simulink model "double_integrator_sim"  (R2023a)
settings: Solver=VariableStepAuto  StartTime=0.0  StopTime=200  FixedStep=0.0001  RelTol=1e-9
values from neighbouring files (symbols this model uses):
  framePeriod_s = 1/frameRate_hz    (= 0.02)    [autocode_setup.m]    (also in setup.m)
undefined symbols (not defined in the file or in its folder): Aircraft, magnitude
libraries: slpidlib x15, simulink x12, dspmathops x2, shared6dof x1, sharedtransform x1
(part 2 of 3)

== system double_integrator_sim/WAYPOINT CONTROLLER1/WP_NAV/Subsystem ==
  Sys_input : Inport
  tar_pos : Inport  Port=2
  max_v_z_mps : Inport  Port=3
  Bus Selector : BusSelector  OutputSignals=StateEstData.aux_ins.ned_pos_m
  Cast To Single : DataTypeConversion  OutDataTypeStr=single  SaturateOnIntegerOverflow=off  RndMeth=Floor
  Selector : Selector  InputPortWidth=3  IndexOptions=Index vector (dialog)  Indices=3  OutputSizes=1
  Selector1 : Selector  InputPortWidth=3  IndexOptions=Index vector (dialog)  Indices=3  OutputSizes=1
  Vertical position controller1 : Subsystem
  ve_z_cmd_mps : Outport
  wires:
  Vertical position controller1/1(ve_z_cmd_mps) -> ve_z_cmd_mps/1  "ve_z_cmd_mps"
  tar_pos/1 -> Selector/1
  Sys_input/1 -> Bus Selector/1
  Bus Selector/1 -> Selector1/1  "<ned_pos_m>"
  Selector1/1 -> Cast To Single/1
  max_v_z_mps/1 -> Vertical position controller1/3(max_v_z_mps)
  Selector/1 -> Vertical position controller1/2(tar_z)
  Cast To Single/1 -> Vertical position controller1/1(cur_alt)

== system double_integrator_sim/WAYPOINT CONTROLLER1/WP_NAV/Vertical position controller ==
  Sys_input : Inport
  max_v_z_mps : Inport  Port=2
  cur_target_pos_m : Inport  Port=3
  Bus Selector6 : BusSelector  OutputSignals=Navigation Filter Data.bfs_ekf.ned_pos_m
  Selector1 : Selector  InputPortWidth=3  IndexOptions=Index vector (dialog)  Indices=3  OutputSizes=1
  select_cur_z : Selector  InputPortWidth=3  IndexOptions=Index vector (dialog)  Indices=3  OutputSizes=1
  vertical_position_controller : Subsystem
  ve_z_cmd_mps : Outport
  wires:
  Sys_input/1 -> Bus Selector6/1
  Bus Selector6/1 -> select_cur_z/1  "<ned_pos_m>"
  vertical_position_controller/1(ve_z_cmd) -> ve_z_cmd_mps/1
  Selector1/1 -> vertical_position_controller/1(target_z_m)  "target_z"
  select_cur_z/1 -> vertical_position_controller/2(cur_z_m)
  cur_target_pos_m/1 -> Selector1/1
  max_v_z_mps/1 -> vertical_position_controller/3(max_v_z_mps)

== system double_integrator_sim/WAYPOINT CONTROLLER1/WP_NAV/heading_controller ==
  Sys_input : Inport
  cur_target_heading_rad : Inport  Port=2
  Bus Selector4 : BusSelector  OutputSignals=Navigation Filter Data.bfs_ekf.heading_rad
  heading_controller : Subsystem
  yaw_rate_cmd_radps : Outport
  wires:
  Sys_input/1 -> Bus Selector4/1
  cur_target_heading_rad/1 -> heading_controller/1(heading_cmd_rad)
  Bus Selector4/1 -> heading_controller/2(<heading_rad>)  "<heading_rad>"
  heading_controller/1(yaw_rate_cmd) -> yaw_rate_cmd_radps/1

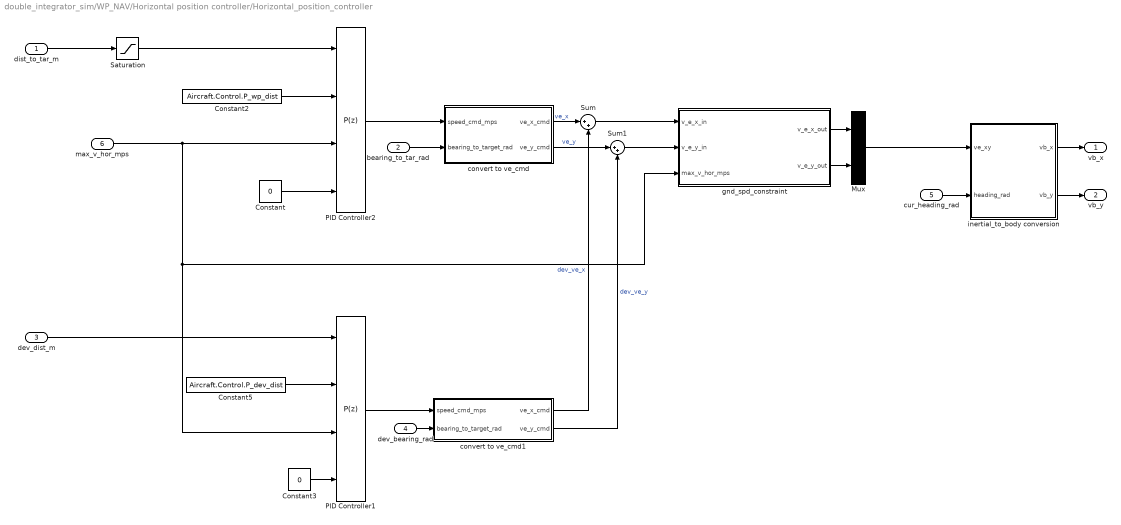
== system double_integrator_sim/WP_NAV/Horizontal position controller/Horizontal_position_controller ==
  dist_to_tar_m : Inport
  bearing_to_tar_rad : Inport  Port=2
  dev_dist_m : Inport  Port=3
  dev_bearing_rad : Inport  Port=4
  cur_heading_rad : Inport  Port=5
  max_v_hor_mps : Inport  Port=6
  Constant : Constant  Value=0  OutDataTypeStr=single
  Constant2 : Constant  Value=Aircraft.Control.P_wp_dist  OutDataTypeStr=single
  Constant3 : Constant  Value=0  OutDataTypeStr=single
  Constant5 : Constant  Value=Aircraft.Control.P_dev_dist  OutDataTypeStr=single
  Mux : Mux  Inputs=2
  PID Controller1 : slpidlib/PID Controller  Controller=P  Form=Parallel  TimeDomain=Discrete-time  UseExternalTs=off  SampleTime=framePeriod_s  IntegratorMethod=Forward Euler  FilterMethod=Forward Euler  ControllerParametersSource=external  P=0.335  I=0.005  UseKiTs=off  D=0  N=100  UseFilter=off  TunerSelectOption=Transfer Function Based (PID Tuner App)  InitialConditionSource=internal  InitialConditionForIntegrator=0  InitialConditionForFilter=0  DifferentiatorICPrevScaledInput=0  ExternalReset=none  TrackingMode=off  Kt=1  LimitOutput=on  SatLimitsSource=external  UpperSaturationLimit=inf  LowerSaturationLimit=-inf  LinearizeAsGain=off  AntiWindupMode=clamping  Kb=1  LimitIntegrator=off  UpperIntegratorSaturationLimit=inf  LowerIntegratorSaturationLimit=-inf  POutMin=[]  POutMax=[]  IOutMin=[]  IOutMax=[]  DOutMin=[]  DOutMax=[]  NOutMin=[]  NOutMax=[]  SumOutMin=[]  SumOutMax=[]  SaturationOutMin=[]  SaturationOutMax=[]  PParamMin=[]  PParamMax=[]  IParamMin=[]  IParamMax=[]  DParamMin=[]  DParamMax=[]  NParamMin=[]  NParamMax=[]  KbParamMin=[]  KbParamMax=[]  KtParamMin=[]  KtParamMax=[]  KbOutMin=[]  KbOutMax=[]  KtOutMin=[]  KtOutMax=[]  IntegratorOutMin=[]  IntegratorOutMax=[]  FilterOutMin=[]  FilterOutMax=[]  SumI1OutMin=[]  SumI1OutMax=[]  SumI2OutMin=[]  SumI2OutMax=[]  SumI3OutMin=[]  SumI3OutMax=[]  SumI4OutMin=[]  SumI4OutMax=[]  SumDOutMin=[]  SumDOutMax=[]  DifferentiatorOutMin=[]  DifferentiatorOutMax=[]  FilterDiffOutCoefMin=[]  FilterDiffOutCoefMax=[]  ReciprocalOutMin=[]  ReciprocalOutMax=[]  SumDenOutMin=[]  SumDenOutMax=[]  SumNumOutMin=[]  SumNumOutMax=[]  DivideOutMin=[]  DivideOutMax=[]  UdiffTsProdOutMin=[]  UdiffTsProdOutMax=[]  NTsProdOutMin=[]  NTsProdOutMax=[]  UintegralTsProdOutMin=[]  UintegralTsProdOutMax=[]  UngainTsProdOutMin=[]  UngainTsProdOutMax=[]  ClampingZeroOutDataTypeStr=Inherit: Inherit via back propagation  ClampingZeroOutMin=[]  ClampingZeroOutMax=[]  FilterDenConstantOutDataTypeStr=Inherit: Inherit via back propagation  FilterDenConstantOutMin=[]  FilterDenConstantOutMax=[]  PCopyOutDataTypeStr=Inherit: Inherit via back propagation  PCopyOutMin=[]  PCopyOutMax=[]  NCopyOutDataTypeStr=Inherit: Inherit via back propagation  NCopyOutMin=[]  NCopyOutMax=[]  IntegratorContinuousStateAttributes=''  IntegratorStateMustResolveToSignalObject=off  IntegratorRTWStateStorageClass=Auto  FilterContinuousStateAttributes=''  FilterStateMustResolveToSignalObject=off  FilterRTWStateStorageClass=Auto  ParallelPVariant=ExternalParameters  IdealPVariant=Disabled  IVariant=Disabled  DVariant=Disabled  IntegratorVariant=Disabled  SatVariant=External  AWVariant=Disabled  PCopyVariant=Disabled  TRVariant=Disabled  FdbkBlocksVariant=Forward  IdealPFdbkVariant=Disabled  SatFdbkVariant=Disabled  DerivativeFilterVariant=Disabled  NVariant=Disabled  NCopyVariant=Disabled_SignalSpec  FilterICVariant=Disabled  IntegratorICVariant=Disabled  ExternalResetVariant=Disabled  TRSumVariant=Passthrough  SumFdbkVariant=Disabled  SumVariant=Passthrough_P  TsampFilterVariant=InternalTs  TsampNgainVariant=Passthrough  TsampIntegralVariant=Disabled_SignalSpec  ExternalSaturationOutDataTypeStr=Inherit: Same as second input
  PID Controller2 : slpidlib/PID Controller  Controller=P  Form=Parallel  TimeDomain=Discrete-time  UseExternalTs=off  SampleTime=framePeriod_s  IntegratorMethod=Forward Euler  FilterMethod=Forward Euler  ControllerParametersSource=external  P=0.335  I=0.005  UseKiTs=off  D=0  N=100  UseFilter=off  TunerSelectOption=Transfer Function Based (PID Tuner App)  InitialConditionSource=internal  InitialConditionForIntegrator=0  InitialConditionForFilter=0  DifferentiatorICPrevScaledInput=0  ExternalReset=none  TrackingMode=off  Kt=1  LimitOutput=on  SatLimitsSource=external  UpperSaturationLimit=inf  LowerSaturationLimit=-inf  LinearizeAsGain=off  AntiWindupMode=clamping  Kb=1  LimitIntegrator=off  UpperIntegratorSaturationLimit=inf  LowerIntegratorSaturationLimit=-inf  POutMin=[]  POutMax=[]  IOutMin=[]  IOutMax=[]  DOutMin=[]  DOutMax=[]  NOutMin=[]  NOutMax=[]  SumOutMin=[]  SumOutMax=[]  SaturationOutMin=[]  SaturationOutMax=[]  PParamMin=[]  PParamMax=[]  IParamMin=[]  IParamMax=[]  DParamMin=[]  DParamMax=[]  NParamMin=[]  NParamMax=[]  KbParamMin=[]  KbParamMax=[]  KtParamMin=[]  KtParamMax=[]  KbOutMin=[]  KbOutMax=[]  KtOutMin=[]  KtOutMax=[]  IntegratorOutMin=[]  IntegratorOutMax=[]  FilterOutMin=[]  FilterOutMax=[]  SumI1OutMin=[]  SumI1OutMax=[]  SumI2OutMin=[]  SumI2OutMax=[]  SumI3OutMin=[]  SumI3OutMax=[]  SumI4OutMin=[]  SumI4OutMax=[]  SumDOutMin=[]  SumDOutMax=[]  DifferentiatorOutMin=[]  DifferentiatorOutMax=[]  FilterDiffOutCoefMin=[]  FilterDiffOutCoefMax=[]  ReciprocalOutMin=[]  ReciprocalOutMax=[]  SumDenOutMin=[]  SumDenOutMax=[]  SumNumOutMin=[]  SumNumOutMax=[]  DivideOutMin=[]  DivideOutMax=[]  UdiffTsProdOutMin=[]  UdiffTsProdOutMax=[]  NTsProdOutMin=[]  NTsProdOutMax=[]  UintegralTsProdOutMin=[]  UintegralTsProdOutMax=[]  UngainTsProdOutMin=[]  UngainTsProdOutMax=[]  ClampingZeroOutDataTypeStr=Inherit: Inherit via back propagation  ClampingZeroOutMin=[]  ClampingZeroOutMax=[]  FilterDenConstantOutDataTypeStr=Inherit: Inherit via back propagation  FilterDenConstantOutMin=[]  FilterDenConstantOutMax=[]  PCopyOutDataTypeStr=Inherit: Inherit via back propagation  PCopyOutMin=[]  PCopyOutMax=[]  NCopyOutDataTypeStr=Inherit: Inherit via back propagation  NCopyOutMin=[]  NCopyOutMax=[]  IntegratorContinuousStateAttributes=''  IntegratorStateMustResolveToSignalObject=off  IntegratorRTWStateStorageClass=Auto  FilterContinuousStateAttributes=''  FilterStateMustResolveToSignalObject=off  FilterRTWStateStorageClass=Auto  ParallelPVariant=ExternalParameters  IdealPVariant=Disabled  IVariant=Disabled  DVariant=Disabled  IntegratorVariant=Disabled  SatVariant=External  AWVariant=Disabled  PCopyVariant=Disabled  TRVariant=Disabled  FdbkBlocksVariant=Forward  IdealPFdbkVariant=Disabled  SatFdbkVariant=Disabled  DerivativeFilterVariant=Disabled  NVariant=Disabled  NCopyVariant=Disabled_SignalSpec  FilterICVariant=Disabled  IntegratorICVariant=Disabled  ExternalResetVariant=Disabled  TRSumVariant=Passthrough  SumFdbkVariant=Disabled  SumVariant=Passthrough_P  TsampFilterVariant=InternalTs  TsampNgainVariant=Passthrough  TsampIntegralVariant=Disabled_SignalSpec  ExternalSaturationOutDataTypeStr=Inherit: Same as second input
  Saturation : Saturate  UpperLimit=1  LowerLimit=0
  Sum : Sum  Inputs=|++
  Sum1 : Sum  Inputs=|++
  convert to ve_cmd : Subsystem
  convert to ve_cmd1 : Subsystem
  "gnd_spd_constraint " : Subsystem
  inertial_to_body conversion : Subsystem
  vb_x : Outport
  vb_y : Outport  Port=2
  wires:
  Constant2/1 -> PID Controller2/2
  bearing_to_tar_rad/1 -> convert to ve_cmd/2(bearing_to_target_rad)
  Mux/1 -> inertial_to_body conversion/1(ve_xy)
  Constant/1 -> PID Controller2/4
  Saturation/1 -> PID Controller2/1
  dist_to_tar_m/1 -> Saturation/1
  cur_heading_rad/1 -> inertial_to_body conversion/2(heading_rad)
  PID Controller2/1 -> convert to ve_cmd/1(speed_cmd_mps)
  inertial_to_body conversion/1(vb_x) -> vb_x/1
  inertial_to_body conversion/2(vb_y) -> vb_y/1
  PID Controller1/1 -> convert to ve_cmd1/1(speed_cmd_mps)
  dev_bearing_rad/1 -> convert to ve_cmd1/2(bearing_to_target_rad)
  dev_dist_m/1 -> PID Controller1/1
  Constant3/1 -> PID Controller1/4
  max_v_hor_mps/1 -> PID Controller1/3, "gnd_spd_constraint "/3(max_v_hor_mps), PID Controller2/3
  convert to ve_cmd/1(ve_x_cmd) -> Sum/1  "ve_x"
  convert to ve_cmd/2(ve_y_cmd) -> Sum1/1  "ve_y"
  convert to ve_cmd1/1(ve_x_cmd) -> Sum/2  "dev_ve_x"
  convert to ve_cmd1/2(ve_y_cmd) -> Sum1/2  "dev_ve_y"
  Sum1/1 -> "gnd_spd_constraint "/2(v_e_y_in)
  Sum/1 -> "gnd_spd_constraint "/1(v_e_x_in)
  "gnd_spd_constraint "/1(v_e_x_out) -> Mux/1
  "gnd_spd_constraint "/2(v_e_y_out) -> Mux/2
  Constant5/1 -> PID Controller1/2

== system double_integrator_sim/WP_NAV/Horizontal position controller/horizontal_error_calculation  ==
  target_pos_m : Inport
  cur_pos_m : Inport  Port=2
  Atan2 : Trigonometry  Operator=atan2
  Cast To Single : DataTypeConversion  OutDataTypeStr=single  SaturateOnIntegerOverflow=off  RndMeth=Floor
  Cast To Single1 : DataTypeConversion  OutDataTypeStr=single  SaturateOnIntegerOverflow=off  RndMeth=Floor
  Demux2 : Demux  Outputs=2
  MatrixMultiply : Product  Multiplication=Matrix(*)
  Selector : Selector  InputPortWidth=3  IndexOptions=Index vector (dialog)  Indices=[1 2]  OutputSizes=1
  Sqrt : Sqrt
  Subtract : Sum  Inputs=+-
  Transpose : Math  Operator=transpose
  dist_to_target_m : Outport
  bearing_to_tar_rad : Outport  Port=2
  wires:
  target_pos_m/1 -> Subtract/1
  cur_pos_m/1 -> Subtract/2
  Selector/1 -> Demux2/1, MatrixMultiply/2, Transpose/1
  Atan2/1 -> Cast To Single1/1
  Subtract/1 -> Selector/1
  Demux2/2 -> Atan2/1
  Transpose/1 -> MatrixMultiply/1
  MatrixMultiply/1 -> Sqrt/1
  Demux2/1 -> Atan2/2
  Sqrt/1 -> Cast To Single/1
  Cast To Single/1 -> dist_to_target_m/1
  Cast To Single1/1 -> bearing_to_tar_rad/1

== system double_integrator_sim/WP_NAV/Subsystem/Vertical position controller1 ==
  cur_alt : Inport
  tar_z : Inport  Port=2
  max_v_z_mps : Inport  Port=3
  Altitude PID : slpidlib/PID Controller  Controller=P  Form=Ideal  TimeDomain=Discrete-time  UseExternalTs=off  SampleTime=framePeriod_s  IntegratorMethod=Forward Euler  FilterMethod=Forward Euler  ControllerParametersSource=external  P=0  I=0  UseKiTs=off  D=0  N=100  UseFilter=off  TunerSelectOption=Frequency Response Based  ZeroCross=off  InitialConditionSource=internal  InitialConditionForIntegrator=0  InitialConditionForFilter=0  DifferentiatorICPrevScaledInput=0  ExternalReset=either  TrackingMode=off  Kt=1  LimitOutput=on  SatLimitsSource=external  UpperSaturationLimit=Aircraft.Control.v_z_max  LowerSaturationLimit=-Aircraft.Control.v_z_max  LinearizeAsGain=on  AntiWindupMode=clamping  Kb=1  LimitIntegrator=off  UpperIntegratorSaturationLimit=inf  LowerIntegratorSaturationLimit=-inf  POutMin=[]  POutMax=[]  IOutMin=[]  IOutMax=[]  DOutMin=[]  DOutMax=[]  NOutMin=[]  NOutMax=[]  SumOutMin=[]  SumOutMax=[]  SaturationOutMin=[]  SaturationOutMax=[]  PParamMin=[]  PParamMax=[]  IParamMin=[]  IParamMax=[]  DParamMin=[]  DParamMax=[]  NParamMin=[]  NParamMax=[]  KbParamMin=[]  KbParamMax=[]  KtParamMin=[]  KtParamMax=[]  KbOutMin=[]  KbOutMax=[]  KtOutMin=[]  KtOutMax=[]  IntegratorOutMin=[]  IntegratorOutMax=[]  FilterOutMin=[]  FilterOutMax=[]  SumI1OutMin=[]  SumI1OutMax=[]  SumI2OutMin=[]  SumI2OutMax=[]  SumI3OutMin=[]  SumI3OutMax=[]  SumI4OutMin=[]  SumI4OutMax=[]  SumDOutMin=[]  SumDOutMax=[]  DifferentiatorOutMin=[]  DifferentiatorOutMax=[]  FilterDiffOutCoefMin=[]  FilterDiffOutCoefMax=[]  ReciprocalOutMin=[]  ReciprocalOutMax=[]  SumDenOutMin=[]  SumDenOutMax=[]  SumNumOutMin=[]  SumNumOutMax=[]  DivideOutMin=[]  DivideOutMax=[]  UdiffTsProdOutMin=[]  UdiffTsProdOutMax=[]  NTsProdOutMin=[]  NTsProdOutMax=[]  UintegralTsProdOutMin=[]  UintegralTsProdOutMax=[]  UngainTsProdOutMin=[]  UngainTsProdOutMax=[]  ClampingZeroOutDataTypeStr=Inherit: Inherit via back propagation  ClampingZeroOutMin=[]  ClampingZeroOutMax=[]  FilterDenConstantOutDataTypeStr=Inherit: Inherit via back propagation  FilterDenConstantOutMin=[]  FilterDenConstantOutMax=[]  PCopyOutDataTypeStr=Inherit: Inherit via back propagation  PCopyOutMin=[]  PCopyOutMax=[]  NCopyOutDataTypeStr=Inherit: Inherit via back propagation  NCopyOutMin=[]  NCopyOutMax=[]  IntegratorContinuousStateAttributes=''  IntegratorStateMustResolveToSignalObject=off  IntegratorRTWStateStorageClass=Auto  FilterContinuousStateAttributes=''  FilterStateMustResolveToSignalObject=off  FilterRTWStateStorageClass=Auto  ParallelPVariant=ExternalParameters  IdealPVariant=Disabled  IVariant=Disabled  DVariant=Disabled  IntegratorVariant=Disabled  SatVariant=External  AWVariant=Disabled  PCopyVariant=Disabled  TRVariant=Disabled  FdbkBlocksVariant=Forward  IdealPFdbkVariant=Disabled  SatFdbkVariant=Disabled  DerivativeFilterVariant=Disabled  NVariant=Disabled  NCopyVariant=Disabled_SignalSpec  FilterICVariant=Disabled  IntegratorICVariant=Disabled  ExternalResetVariant=Disabled  TRSumVariant=Passthrough  SumFdbkVariant=Disabled  SumVariant=Passthrough_P  TsampFilterVariant=InternalTs  TsampNgainVariant=Passthrough  TsampIntegralVariant=Disabled_SignalSpec  ExternalSaturationOutDataTypeStr=Inherit: Same as second input
  Constant3 : Constant  Value=0.1  OutDataTypeStr=single
  Gain : Gain  Gain=-1
  Scope : Scope  NumInputPorts=3
  Sum3 : Sum  Inputs=|+-
  ve_z_cmd_mps : Outport
  wires:
  Altitude PID/1 -> Scope/3, ve_z_cmd_mps/1
  tar_z/1 -> Scope/1, Sum3/1  "target_z"
  cur_alt/1 -> Scope/2, Sum3/2
  Sum3/1 -> Altitude PID/1
  Constant3/1 -> Altitude PID/2
  max_v_z_mps/1 -> Gain/1, Altitude PID/3
  Gain/1 -> Altitude PID/4

== system double_integrator_sim/WP_NAV/Vertical position controller/vertical_position_controller ==
  target_z_m : Inport
  cur_z_m : Inport  Port=2
  max_v_z_mps : Inport  Port=3
  Altitude PID : slpidlib/PID Controller  Controller=PI  Form=Ideal  TimeDomain=Discrete-time  UseExternalTs=off  SampleTime=framePeriod_s  IntegratorMethod=Forward Euler  FilterMethod=Forward Euler  ControllerParametersSource=external  P=0  I=0  UseKiTs=off  D=0  N=100  UseFilter=off  TunerSelectOption=Frequency Response Based  ZeroCross=off  InitialConditionSource=internal  InitialConditionForIntegrator=0  InitialConditionForFilter=0  DifferentiatorICPrevScaledInput=0  ExternalReset=none  TrackingMode=off  Kt=1  LimitOutput=on  SatLimitsSource=external  UpperSaturationLimit=Aircraft.Control.v_z_up_max  LowerSaturationLimit=-Aircraft.Control.v_z_down_max  LinearizeAsGain=on  AntiWindupMode=clamping  Kb=1  POutMin=[]  POutMax=[]  IOutMin=[]  IOutMax=[]  DOutMin=[]  DOutMax=[]  NOutMin=[]  NOutMax=[]  SumOutMin=[]  SumOutMax=[]  SaturationOutMin=[]  SaturationOutMax=[]  PParamMin=[]  PParamMax=[]  IParamMin=[]  IParamMax=[]  DParamMin=[]  DParamMax=[]  NParamMin=[]  NParamMax=[]  KbParamMin=[]  KbParamMax=[]  KtParamMin=[]  KtParamMax=[]  KbOutMin=[]  KbOutMax=[]  KtOutMin=[]  KtOutMax=[]  IntegratorOutMin=[]  IntegratorOutMax=[]  FilterOutMin=[]  FilterOutMax=[]  SumI1OutMin=[]  SumI1OutMax=[]  SumI2OutMin=[]  SumI2OutMax=[]  SumI3OutMin=[]  SumI3OutMax=[]  SumI4OutMin=[]  SumI4OutMax=[]  SumDOutMin=[]  SumDOutMax=[]  DifferentiatorOutMin=[]  DifferentiatorOutMax=[]  FilterDiffOutCoefMin=[]  FilterDiffOutCoefMax=[]  ReciprocalOutMin=[]  ReciprocalOutMax=[]  SumDenOutMin=[]  SumDenOutMax=[]  SumNumOutMin=[]  SumNumOutMax=[]  DivideOutMin=[]  DivideOutMax=[]  UdiffTsProdOutMin=[]  UdiffTsProdOutMax=[]  NTsProdOutMin=[]  NTsProdOutMax=[]  UintegralTsProdOutMin=[]  UintegralTsProdOutMax=[]  UngainTsProdOutMin=[]  UngainTsProdOutMax=[]  IntegratorContinuousStateAttributes=''  IntegratorStateMustResolveToSignalObject=off  IntegratorRTWStateStorageClass=Auto  FilterContinuousStateAttributes=''  FilterStateMustResolveToSignalObject=off  FilterRTWStateStorageClass=Auto  ParallelPVariant=Passthrough  IdealPVariant=ExternalParameters  IVariant=ExternalParameters  DVariant=Disabled  IntegratorVariant=Discrete  SatVariant=External  AWVariant=DiscClampingIdeal  PCopyVariant=ExternalParamsIdeal  TRVariant=Disabled  FdbkBlocksVariant=Forward  IdealPFdbkVariant=Disabled  SatFdbkVariant=Disabled  DerivativeFilterVariant=Disabled  NVariant=Disabled  NCopyVariant=Disabled_SignalSpec  FilterICVariant=Disabled  IntegratorICVariant=InternalICs  ExternalResetVariant=Disabled  TRSumVariant=Passthrough  SumFdbkVariant=Disabled  SumVariant=Sum_PI  TsampFilterVariant=InternalTs  TsampNgainVariant=Passthrough  TsampIntegralVariant=Passthrough  ExternalSaturationOutDataTypeStr=Inherit: Same as second input  aMode=0
  Constant : Constant  Value=Aircraft.Control.v_z_up_max  OutDataTypeStr=single
  Constant1 : Constant  Value=Aircraft.Control.v_z_down_max  OutDataTypeStr=single
  Gain : Gain  Gain=-1
  Min : MinMax  Inputs=2
  P_alt : Constant  Value=Aircraft.Control.P_alt  OutDataTypeStr=single
  P_alt1 : Constant  Value=Aircraft.Control.I_alt  OutDataTypeStr=single
  Sum3 : Sum  Inputs=|+-
  ve_z_cmd : Outport
  wires:
  P_alt/1 -> Altitude PID/2
  Sum3/1 -> Altitude PID/1
  max_v_z_mps/1 -> Min/1
  Constant/1 -> Min/2
  Constant1/1 -> Altitude PID/4
  Min/1 -> Gain/1
  Gain/1 -> Altitude PID/5
  P_alt1/1 -> Altitude PID/3
  Altitude PID/1 -> ve_z_cmd/1
  target_z_m/1 -> Sum3/1
  cur_z_m/1 -> Sum3/2

== system double_integrator_sim/WP_NAV/heading_controller/heading_controller ==
  heading_cmd_rad : Inport
  <heading_rad> : Inport  Port=2
  D_heading : Constant  Value=Aircraft.Control.D_heading  OutDataTypeStr=single
  Discrete Derivative : simulink/Discrete/Discrete Derivative  gainval=1.0  ICPrevScaledInput=0.0  OutMin=[]  OutMax=[]  OutDataType=fixdt(1, 16)  OutScaling=2^-10  DoSatur=off
  I_heading : Constant  Value=Aircraft.Control.I_heading  OutDataTypeStr=single
  PID Controller2 : slpidlib/PID Controller  Controller=PI  Form=Ideal  TimeDomain=Discrete-time  UseExternalTs=off  SampleTime=framePeriod_s  IntegratorMethod=Forward Euler  FilterMethod=Forward Euler  ControllerParametersSource=external  P=1.85  I=0.01  UseKiTs=off  D=0  N=100  UseFilter=off  TunerSelectOption=Transfer Function Based (PID Tuner App)  InitialConditionSource=internal  InitialConditionForIntegrator=0  InitialConditionForFilter=0  DifferentiatorICPrevScaledInput=0  ExternalReset=none  TrackingMode=off  Kt=1  LimitOutput=on  SatLimitsSource=internal  UpperSaturationLimit=inf  LowerSaturationLimit=-inf  LinearizeAsGain=on  AntiWindupMode=clamping  Kb=2  POutMin=[]  POutMax=[]  IOutMin=[]  IOutMax=[]  DOutMin=[]  DOutMax=[]  NOutMin=[]  NOutMax=[]  SumOutMin=[]  SumOutMax=[]  SaturationOutMin=[]  SaturationOutMax=[]  PParamMin=[]  PParamMax=[]  IParamMin=[]  IParamMax=[]  DParamMin=[]  DParamMax=[]  NParamMin=[]  NParamMax=[]  KbParamMin=[]  KbParamMax=[]  KtParamMin=[]  KtParamMax=[]  KbOutMin=[]  KbOutMax=[]  KtOutMin=[]  KtOutMax=[]  IntegratorOutMin=[]  IntegratorOutMax=[]  FilterOutMin=[]  FilterOutMax=[]  SumI1OutMin=[]  SumI1OutMax=[]  SumI2OutMin=[]  SumI2OutMax=[]  SumI3OutMin=[]  SumI3OutMax=[]  SumI4OutMin=[]  SumI4OutMax=[]  SumDOutMin=[]  SumDOutMax=[]  DifferentiatorOutMin=[]  DifferentiatorOutMax=[]  FilterDiffOutCoefMin=[]  FilterDiffOutCoefMax=[]  ReciprocalOutMin=[]  ReciprocalOutMax=[]  SumDenOutMin=[]  SumDenOutMax=[]  SumNumOutMin=[]  SumNumOutMax=[]  DivideOutMin=[]  DivideOutMax=[]  UdiffTsProdOutMin=[]  UdiffTsProdOutMax=[]  NTsProdOutMin=[]  NTsProdOutMax=[]  UintegralTsProdOutMin=[]  UintegralTsProdOutMax=[]  UngainTsProdOutMin=[]  UngainTsProdOutMax=[]  IntegratorContinuousStateAttributes=''  IntegratorStateMustResolveToSignalObject=off  IntegratorRTWStateStorageClass=Auto  FilterContinuousStateAttributes=''  FilterStateMustResolveToSignalObject=off  FilterRTWStateStorageClass=Auto  ParallelPVariant=Passthrough  IdealPVariant=ExternalParameters  IVariant=ExternalParameters  DVariant=Disabled  IntegratorVariant=Discrete  SatVariant=Enabled  AWVariant=DiscClampingIdeal  PCopyVariant=ExternalParamsIdeal  TRVariant=Disabled  FdbkBlocksVariant=Forward  IdealPFdbkVariant=Disabled  SatFdbkVariant=Disabled  DerivativeFilterVariant=Disabled  NVariant=Disabled  NCopyVariant=Disabled_SignalSpec  FilterICVariant=Disabled  IntegratorICVariant=InternalICs  ExternalResetVariant=Disabled  TRSumVariant=Passthrough  SumFdbkVariant=Disabled  SumVariant=Sum_PI  TsampFilterVariant=InternalTs  TsampNgainVariant=Passthrough  TsampIntegralVariant=Passthrough  ExternalSaturationOutDataTypeStr=Inherit: Same as second input  aMode=0
  P_heading : Constant  Value=Aircraft.Control.P_heading  OutDataTypeStr=single
  Product : Product
  Saturation : Saturate  UpperLimit=Aircraft.Control.yaw_rate_max  LowerLimit=-Aircraft.Control.yaw_rate_max
  Sum : Sum  Inputs=|+-
  heading_error : Subsystem
  yaw_rate_cmd : Outport
  wires:
  P_heading/1 -> PID Controller2/2
  heading_cmd_rad/1 -> heading_error/1(heading_cmd_rad)
  I_heading/1 -> PID Controller2/3
  <heading_rad>/1 -> Discrete Derivative/1, heading_error/2(heading_rad)
  Saturation/1 -> yaw_rate_cmd/1
  heading_error/1(heading_error_rad) -> PID Controller2/1
  Discrete Derivative/1 -> Product/1
  D_heading/1 -> Product/2
  PID Controller2/1 -> Sum/1
  Sum/1 -> Saturation/1
  Product/1 -> Sum/2

== system double_integrator_sim/POS_HOLD CONTROLLER/Horizontal speed controller/Subsystem/roll_D_DLPF ==
  raw_val : Inport
  freq_cut : Inport  Port=2
  Cast To Single : DataTypeConversion  OutDataTypeStr=single  SaturateOnIntegerOverflow=off  RndMeth=Floor
  Constant : Constant  Value=50  OutDataTypeStr=single
  MATLAB Function : MATLAB Function  TreatAsAtomicUnit=on
  Unit Delay : UnitDelay  SampleTime=-1  HasFrameUpgradeWarning=on
  filtered_val : Outport
  wires:
  freq_cut/1 -> MATLAB Function/3(freq_cut)
  MATLAB Function/1(filtered_val) -> Unit Delay/1, filtered_val/1
  Unit Delay/1 -> Cast To Single/1
  raw_val/1 -> MATLAB Function/2(raw_val)
  Constant/1 -> MATLAB Function/4(samp_freq)
  Cast To Single/1 -> MATLAB Function/1(prev_val)

== system double_integrator_sim/POS_HOLD CONTROLLER/Horizontal speed controller/Subsystem/roll_D_DLPF1 ==
  raw_val : Inport
  freq_cut : Inport  Port=2
  Cast To Single : DataTypeConversion  OutDataTypeStr=single  SaturateOnIntegerOverflow=off  RndMeth=Floor
  Constant : Constant  Value=50  OutDataTypeStr=single
  MATLAB Function : MATLAB Function  TreatAsAtomicUnit=on
  Unit Delay : UnitDelay  SampleTime=-1  HasFrameUpgradeWarning=on
  filtered_val : Outport
  wires:
  Constant/1 -> MATLAB Function/4(samp_freq)
  raw_val/1 -> MATLAB Function/2(raw_val)
  Unit Delay/1 -> Cast To Single/1
  MATLAB Function/1(filtered_val) -> filtered_val/1, Unit Delay/1
  freq_cut/1 -> MATLAB Function/3(freq_cut)
  Cast To Single/1 -> MATLAB Function/1(prev_val)

== system double_integrator_sim/POS_HOLD CONTROLLER/Horizontal speed controller/Subsystem1/roll_D_DLPF ==
  raw_val : Inport
  freq_cut : Inport  Port=2
  Cast To Single : DataTypeConversion  OutDataTypeStr=single  SaturateOnIntegerOverflow=off  RndMeth=Floor
  Constant : Constant  Value=50  OutDataTypeStr=single
  MATLAB Function : MATLAB Function  TreatAsAtomicUnit=on
  Unit Delay : UnitDelay  SampleTime=-1  HasFrameUpgradeWarning=on
  filtered_val : Outport
  wires:
  freq_cut/1 -> MATLAB Function/3(freq_cut)
  MATLAB Function/1(filtered_val) -> Unit Delay/1, filtered_val/1
  Unit Delay/1 -> Cast To Single/1
  raw_val/1 -> MATLAB Function/2(raw_val)
  Constant/1 -> MATLAB Function/4(samp_freq)
  Cast To Single/1 -> MATLAB Function/1(prev_val)

== system double_integrator_sim/POS_HOLD CONTROLLER/Horizontal speed controller/Subsystem1/roll_D_DLPF1 ==
  raw_val : Inport
  freq_cut : Inport  Port=2
  Cast To Single : DataTypeConversion  OutDataTypeStr=single  SaturateOnIntegerOverflow=off  RndMeth=Floor
  Constant : Constant  Value=50  OutDataTypeStr=single
  MATLAB Function : MATLAB Function  TreatAsAtomicUnit=on
  Unit Delay : UnitDelay  SampleTime=-1  HasFrameUpgradeWarning=on
  filtered_val : Outport
  wires:
  Constant/1 -> MATLAB Function/4(samp_freq)
  raw_val/1 -> MATLAB Function/2(raw_val)
  Unit Delay/1 -> Cast To Single/1
  MATLAB Function/1(filtered_val) -> filtered_val/1, Unit Delay/1
  freq_cut/1 -> MATLAB Function/3(freq_cut)
  Cast To Single/1 -> MATLAB Function/1(prev_val)

== system double_integrator_sim/POS_HOLD CONTROLLER/Horizontal speed controller/zero_vel_handling/Horizontal position controller ==
  cur_target_pos_m : Inport
  cur_pos_m : Inport  Port=2
  cur_heading_rad : Inport  Port=3
  Horizontal_position_controller : Subsystem
  "horizontal_error_calculation " : Subsystem
  vb_x_cmd_mps : Outport
  vb_y_cmd_mps : Outport  Port=2
  wires:
  Horizontal_position_controller/1(vb_x) -> vb_x_cmd_mps/1
  Horizontal_position_controller/2(vb_y) -> vb_y_cmd_mps/1
  "horizontal_error_calculation "/1(dist_to_target_m) -> Horizontal_position_controller/1(dist_to_tar_m)
  "horizontal_error_calculation "/2(bearing_to_tar_rad) -> Horizontal_position_controller/2(bearing_to_tar_rad)
  cur_target_pos_m/1 -> "horizontal_error_calculation "/1(target_pos_m)
  cur_pos_m/1 -> "horizontal_error_calculation "/2(cur_pos_m)
  cur_heading_rad/1 -> Horizontal_position_controller/3(cur_heading_rad)

== system double_integrator_sim/POS_HOLD CONTROLLER/Horizontal speed controller/zero_vel_handling/set_tar_pos when vel_cmd == 0 ==
  pos_xy_m : Inport
  Enable : EnablePort
  target_pos_xy_m : Outport
  wires:
  pos_xy_m/1 -> target_pos_xy_m/1

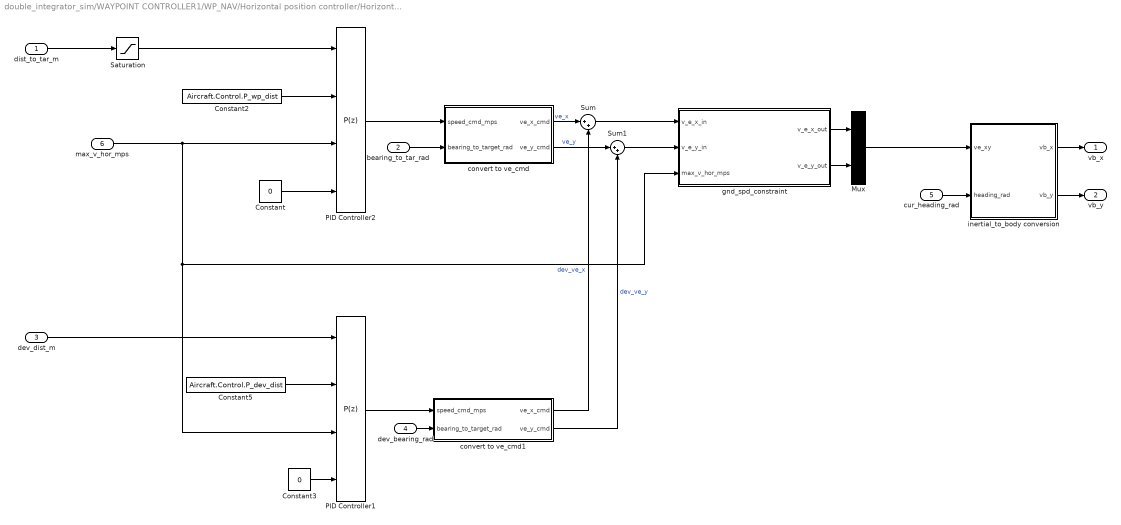
== system double_integrator_sim/WAYPOINT CONTROLLER1/WP_NAV/Horizontal position controller/Horizontal_position_controller ==
  dist_to_tar_m : Inport
  bearing_to_tar_rad : Inport  Port=2
  dev_dist_m : Inport  Port=3
  dev_bearing_rad : Inport  Port=4
  cur_heading_rad : Inport  Port=5
  max_v_hor_mps : Inport  Port=6
  Constant : Constant  Value=0  OutDataTypeStr=single
  Constant2 : Constant  Value=Aircraft.Control.P_wp_dist  OutDataTypeStr=single
  Constant3 : Constant  Value=0  OutDataTypeStr=single
  Constant5 : Constant  Value=Aircraft.Control.P_dev_dist  OutDataTypeStr=single
  Mux : Mux  Inputs=2
  PID Controller1 : slpidlib/PID Controller  Controller=P  Form=Parallel  TimeDomain=Discrete-time  UseExternalTs=off  SampleTime=framePeriod_s  IntegratorMethod=Forward Euler  FilterMethod=Forward Euler  ControllerParametersSource=external  P=0.335  I=0.005  UseKiTs=off  D=0  N=100  UseFilter=off  TunerSelectOption=Transfer Function Based (PID Tuner App)  InitialConditionSource=internal  InitialConditionForIntegrator=0  InitialConditionForFilter=0  DifferentiatorICPrevScaledInput=0  ExternalReset=none  TrackingMode=off  Kt=1  LimitOutput=on  SatLimitsSource=external  UpperSaturationLimit=inf  LowerSaturationLimit=-inf  LinearizeAsGain=off  AntiWindupMode=clamping  Kb=1  POutMin=[]  POutMax=[]  IOutMin=[]  IOutMax=[]  DOutMin=[]  DOutMax=[]  NOutMin=[]  NOutMax=[]  SumOutMin=[]  SumOutMax=[]  SaturationOutMin=[]  SaturationOutMax=[]  PParamMin=[]  PParamMax=[]  IParamMin=[]  IParamMax=[]  DParamMin=[]  DParamMax=[]  NParamMin=[]  NParamMax=[]  KbParamMin=[]  KbParamMax=[]  KtParamMin=[]  KtParamMax=[]  KbOutMin=[]  KbOutMax=[]  KtOutMin=[]  KtOutMax=[]  IntegratorOutMin=[]  IntegratorOutMax=[]  FilterOutMin=[]  FilterOutMax=[]  SumI1OutMin=[]  SumI1OutMax=[]  SumI2OutMin=[]  SumI2OutMax=[]  SumI3OutMin=[]  SumI3OutMax=[]  SumI4OutMin=[]  SumI4OutMax=[]  SumDOutMin=[]  SumDOutMax=[]  DifferentiatorOutMin=[]  DifferentiatorOutMax=[]  FilterDiffOutCoefMin=[]  FilterDiffOutCoefMax=[]  ReciprocalOutMin=[]  ReciprocalOutMax=[]  SumDenOutMin=[]  SumDenOutMax=[]  SumNumOutMin=[]  SumNumOutMax=[]  DivideOutMin=[]  DivideOutMax=[]  UdiffTsProdOutMin=[]  UdiffTsProdOutMax=[]  NTsProdOutMin=[]  NTsProdOutMax=[]  UintegralTsProdOutMin=[]  UintegralTsProdOutMax=[]  UngainTsProdOutMin=[]  UngainTsProdOutMax=[]  IntegratorContinuousStateAttributes=''  IntegratorStateMustResolveToSignalObject=off  IntegratorRTWStateStorageClass=Auto  FilterContinuousStateAttributes=''  FilterStateMustResolveToSignalObject=off  FilterRTWStateStorageClass=Auto  ParallelPVariant=ExternalParameters  IdealPVariant=Disabled  IVariant=Disabled  DVariant=Disabled  IntegratorVariant=Disabled  SatVariant=External  AWVariant=Disabled  PCopyVariant=Disabled  TRVariant=Disabled  FdbkBlocksVariant=Forward  IdealPFdbkVariant=Disabled  SatFdbkVariant=Disabled  DerivativeFilterVariant=Disabled  NVariant=Disabled  NCopyVariant=Disabled_SignalSpec  FilterICVariant=Disabled  IntegratorICVariant=Disabled  ExternalResetVariant=Disabled  TRSumVariant=Passthrough  SumFdbkVariant=Disabled  SumVariant=Passthrough_P  TsampFilterVariant=InternalTs  TsampNgainVariant=Passthrough  TsampIntegralVariant=Disabled_SignalSpec  ExternalSaturationOutDataTypeStr=Inherit: Same as second input  aMode=0
  PID Controller2 : slpidlib/PID Controller  Controller=P  Form=Parallel  TimeDomain=Discrete-time  UseExternalTs=off  SampleTime=framePeriod_s  IntegratorMethod=Forward Euler  FilterMethod=Forward Euler  ControllerParametersSource=external  P=0.335  I=0.005  UseKiTs=off  D=0  N=100  UseFilter=off  TunerSelectOption=Transfer Function Based (PID Tuner App)  InitialConditionSource=internal  InitialConditionForIntegrator=0  InitialConditionForFilter=0  DifferentiatorICPrevScaledInput=0  ExternalReset=none  TrackingMode=off  Kt=1  LimitOutput=on  SatLimitsSource=external  UpperSaturationLimit=inf  LowerSaturationLimit=-inf  LinearizeAsGain=off  AntiWindupMode=clamping  Kb=1  POutMin=[]  POutMax=[]  IOutMin=[]  IOutMax=[]  DOutMin=[]  DOutMax=[]  NOutMin=[]  NOutMax=[]  SumOutMin=[]  SumOutMax=[]  SaturationOutMin=[]  SaturationOutMax=[]  PParamMin=[]  PParamMax=[]  IParamMin=[]  IParamMax=[]  DParamMin=[]  DParamMax=[]  NParamMin=[]  NParamMax=[]  KbParamMin=[]  KbParamMax=[]  KtParamMin=[]  KtParamMax=[]  KbOutMin=[]  KbOutMax=[]  KtOutMin=[]  KtOutMax=[]  IntegratorOutMin=[]  IntegratorOutMax=[]  FilterOutMin=[]  FilterOutMax=[]  SumI1OutMin=[]  SumI1OutMax=[]  SumI2OutMin=[]  SumI2OutMax=[]  SumI3OutMin=[]  SumI3OutMax=[]  SumI4OutMin=[]  SumI4OutMax=[]  SumDOutMin=[]  SumDOutMax=[]  DifferentiatorOutMin=[]  DifferentiatorOutMax=[]  FilterDiffOutCoefMin=[]  FilterDiffOutCoefMax=[]  ReciprocalOutMin=[]  ReciprocalOutMax=[]  SumDenOutMin=[]  SumDenOutMax=[]  SumNumOutMin=[]  SumNumOutMax=[]  DivideOutMin=[]  DivideOutMax=[]  UdiffTsProdOutMin=[]  UdiffTsProdOutMax=[]  NTsProdOutMin=[]  NTsProdOutMax=[]  UintegralTsProdOutMin=[]  UintegralTsProdOutMax=[]  UngainTsProdOutMin=[]  UngainTsProdOutMax=[]  IntegratorContinuousStateAttributes=''  IntegratorStateMustResolveToSignalObject=off  IntegratorRTWStateStorageClass=Auto  FilterContinuousStateAttributes=''  FilterStateMustResolveToSignalObject=off  FilterRTWStateStorageClass=Auto  ParallelPVariant=ExternalParameters  IdealPVariant=Disabled  IVariant=Disabled  DVariant=Disabled  IntegratorVariant=Disabled  SatVariant=External  AWVariant=Disabled  PCopyVariant=Disabled  TRVariant=Disabled  FdbkBlocksVariant=Forward  IdealPFdbkVariant=Disabled  SatFdbkVariant=Disabled  DerivativeFilterVariant=Disabled  NVariant=Disabled  NCopyVariant=Disabled_SignalSpec  FilterICVariant=Disabled  IntegratorICVariant=Disabled  ExternalResetVariant=Disabled  TRSumVariant=Passthrough  SumFdbkVariant=Disabled  SumVariant=Passthrough_P  TsampFilterVariant=InternalTs  TsampNgainVariant=Passthrough  TsampIntegralVariant=Disabled_SignalSpec  ExternalSaturationOutDataTypeStr=Inherit: Same as second input  aMode=0
  Saturation : Saturate  UpperLimit=1  LowerLimit=0
  Sum : Sum  Inputs=|++
  Sum1 : Sum  Inputs=|++
  convert to ve_cmd : Subsystem
  convert to ve_cmd1 : Subsystem
  "gnd_spd_constraint " : Subsystem
  inertial_to_body conversion : Subsystem
  vb_x : Outport
  vb_y : Outport  Port=2
  wires:
  Constant2/1 -> PID Controller2/2
  bearing_to_tar_rad/1 -> convert to ve_cmd/2(bearing_to_target_rad)
  Mux/1 -> inertial_to_body conversion/1(ve_xy)
  Constant/1 -> PID Controller2/4
  Saturation/1 -> PID Controller2/1
  dist_to_tar_m/1 -> Saturation/1
  cur_heading_rad/1 -> inertial_to_body conversion/2(heading_rad)
  PID Controller2/1 -> convert to ve_cmd/1(speed_cmd_mps)
  inertial_to_body conversion/1(vb_x) -> vb_x/1
  inertial_to_body conversion/2(vb_y) -> vb_y/1
  PID Controller1/1 -> convert to ve_cmd1/1(speed_cmd_mps)
  dev_bearing_rad/1 -> convert to ve_cmd1/2(bearing_to_target_rad)
  dev_dist_m/1 -> PID Controller1/1
  Constant3/1 -> PID Controller1/4
  max_v_hor_mps/1 -> PID Controller1/3, "gnd_spd_constraint "/3(max_v_hor_mps), PID Controller2/3
  convert to ve_cmd/1(ve_x_cmd) -> Sum/1  "ve_x"
  convert to ve_cmd/2(ve_y_cmd) -> Sum1/1  "ve_y"
  convert to ve_cmd1/1(ve_x_cmd) -> Sum/2  "dev_ve_x"
  convert to ve_cmd1/2(ve_y_cmd) -> Sum1/2  "dev_ve_y"
  Sum1/1 -> "gnd_spd_constraint "/2(v_e_y_in)
  Sum/1 -> "gnd_spd_constraint "/1(v_e_x_in)
  "gnd_spd_constraint "/1(v_e_x_out) -> Mux/1
  "gnd_spd_constraint "/2(v_e_y_out) -> Mux/2
  Constant5/1 -> PID Controller1/2

== system double_integrator_sim/WAYPOINT CONTROLLER1/WP_NAV/Horizontal position controller/horizontal_error_calculation  ==
  target_pos_m : Inport
  cur_pos_m : Inport  Port=2
  Atan2 : Trigonometry  Operator=atan2
  Demux2 : Demux  Outputs=2
  MatrixMultiply : Product  Multiplication=Matrix(*)
  Selector : Selector  InputPortWidth=3  IndexOptions=Index vector (dialog)  Indices=[1 2]  OutputSizes=1
  Sqrt : Sqrt
  Subtract : Sum  Inputs=+-
  Transpose : Math  Operator=transpose
  dist_to_target_m : Outport
  bearing_to_tar_rad : Outport  Port=2
  wires:
  target_pos_m/1 -> Subtract/1
  cur_pos_m/1 -> Subtract/2
  Selector/1 -> Demux2/1, MatrixMultiply/2, Transpose/1
  Atan2/1 -> bearing_to_tar_rad/1
  Subtract/1 -> Selector/1
  Demux2/2 -> Atan2/1
  Transpose/1 -> MatrixMultiply/1
  MatrixMultiply/1 -> Sqrt/1
  Demux2/1 -> Atan2/2
  Sqrt/1 -> dist_to_target_m/1

== system double_integrator_sim/WAYPOINT CONTROLLER1/WP_NAV/Subsystem/Vertical position controller1 ==
  cur_alt : Inport
  tar_z : Inport  Port=2
  max_v_z_mps : Inport  Port=3
  Altitude PID : slpidlib/PID Controller  Controller=P  Form=Ideal  TimeDomain=Discrete-time  UseExternalTs=off  SampleTime=framePeriod_s  IntegratorMethod=Forward Euler  FilterMethod=Forward Euler  ControllerParametersSource=external  P=0  I=0  UseKiTs=off  D=0  N=100  UseFilter=off  TunerSelectOption=Frequency Response Based  ZeroCross=off  InitialConditionSource=internal  InitialConditionForIntegrator=0  InitialConditionForFilter=0  DifferentiatorICPrevScaledInput=0  ExternalReset=either  TrackingMode=off  Kt=1  LimitOutput=on  SatLimitsSource=external  UpperSaturationLimit=Aircraft.Control.v_z_max  LowerSaturationLimit=-Aircraft.Control.v_z_max  LinearizeAsGain=on  AntiWindupMode=clamping  Kb=1  POutMin=[]  POutMax=[]  IOutMin=[]  IOutMax=[]  DOutMin=[]  DOutMax=[]  NOutMin=[]  NOutMax=[]  SumOutMin=[]  SumOutMax=[]  SaturationOutMin=[]  SaturationOutMax=[]  PParamMin=[]  PParamMax=[]  IParamMin=[]  IParamMax=[]  DParamMin=[]  DParamMax=[]  NParamMin=[]  NParamMax=[]  KbParamMin=[]  KbParamMax=[]  KtParamMin=[]  KtParamMax=[]  KbOutMin=[]  KbOutMax=[]  KtOutMin=[]  KtOutMax=[]  IntegratorOutMin=[]  IntegratorOutMax=[]  FilterOutMin=[]  FilterOutMax=[]  SumI1OutMin=[]  SumI1OutMax=[]  SumI2OutMin=[]  SumI2OutMax=[]  SumI3OutMin=[]  SumI3OutMax=[]  SumI4OutMin=[]  SumI4OutMax=[]  SumDOutMin=[]  SumDOutMax=[]  DifferentiatorOutMin=[]  DifferentiatorOutMax=[]  FilterDiffOutCoefMin=[]  FilterDiffOutCoefMax=[]  ReciprocalOutMin=[]  ReciprocalOutMax=[]  SumDenOutMin=[]  SumDenOutMax=[]  SumNumOutMin=[]  SumNumOutMax=[]  DivideOutMin=[]  DivideOutMax=[]  UdiffTsProdOutMin=[]  UdiffTsProdOutMax=[]  NTsProdOutMin=[]  NTsProdOutMax=[]  UintegralTsProdOutMin=[]  UintegralTsProdOutMax=[]  UngainTsProdOutMin=[]  UngainTsProdOutMax=[]  IntegratorContinuousStateAttributes=''  IntegratorStateMustResolveToSignalObject=off  IntegratorRTWStateStorageClass=Auto  FilterContinuousStateAttributes=''  FilterStateMustResolveToSignalObject=off  FilterRTWStateStorageClass=Auto  ParallelPVariant=ExternalParameters  IdealPVariant=Disabled  IVariant=Disabled  DVariant=Disabled  IntegratorVariant=Disabled  SatVariant=External  AWVariant=Disabled  PCopyVariant=Disabled  TRVariant=Disabled  FdbkBlocksVariant=Forward  IdealPFdbkVariant=Disabled  SatFdbkVariant=Disabled  DerivativeFilterVariant=Disabled  NVariant=Disabled  NCopyVariant=Disabled_SignalSpec  FilterICVariant=Disabled  IntegratorICVariant=Disabled  ExternalResetVariant=Disabled  TRSumVariant=Passthrough  SumFdbkVariant=Disabled  SumVariant=Passthrough_P  TsampFilterVariant=InternalTs  TsampNgainVariant=Passthrough  TsampIntegralVariant=Disabled_SignalSpec  ExternalSaturationOutDataTypeStr=Inherit: Same as second input  aMode=0
  Constant3 : Constant  Value=Aircraft.Control.P_alt  OutDataTypeStr=single
  Gain : Gain  Gain=-1
  Sum3 : Sum  Inputs=|+-
  ve_z_cmd_mps : Outport
  wires:
  Altitude PID/1 -> ve_z_cmd_mps/1
  tar_z/1 -> Sum3/1  "target_z"
  cur_alt/1 -> Sum3/2
  Sum3/1 -> Altitude PID/1
  Constant3/1 -> Altitude PID/2
  max_v_z_mps/1 -> Gain/1, Altitude PID/3
  Gain/1 -> Altitude PID/4

== system double_integrator_sim/WAYPOINT CONTROLLER1/WP_NAV/Vertical position controller/vertical_position_controller ==
  target_z_m : Inport
  cur_z_m : Inport  Port=2
  max_v_z_mps : Inport  Port=3
  Altitude PID : slpidlib/PID Controller  Controller=PI  Form=Ideal  TimeDomain=Discrete-time  UseExternalTs=off  SampleTime=framePeriod_s  IntegratorMethod=Forward Euler  FilterMethod=Forward Euler  ControllerParametersSource=external  P=0  I=0  UseKiTs=off  D=0  N=100  UseFilter=off  TunerSelectOption=Frequency Response Based  ZeroCross=off  InitialConditionSource=internal  InitialConditionForIntegrator=0  InitialConditionForFilter=0  DifferentiatorICPrevScaledInput=0  ExternalReset=none  TrackingMode=off  Kt=1  LimitOutput=on  SatLimitsSource=external  UpperSaturationLimit=Aircraft.Control.v_z_up_max  LowerSaturationLimit=-Aircraft.Control.v_z_down_max  LinearizeAsGain=on  AntiWindupMode=clamping  Kb=1  POutMin=[]  POutMax=[]  IOutMin=[]  IOutMax=[]  DOutMin=[]  DOutMax=[]  NOutMin=[]  NOutMax=[]  SumOutMin=[]  SumOutMax=[]  SaturationOutMin=[]  SaturationOutMax=[]  PParamMin=[]  PParamMax=[]  IParamMin=[]  IParamMax=[]  DParamMin=[]  DParamMax=[]  NParamMin=[]  NParamMax=[]  KbParamMin=[]  KbParamMax=[]  KtParamMin=[]  KtParamMax=[]  KbOutMin=[]  KbOutMax=[]  KtOutMin=[]  KtOutMax=[]  IntegratorOutMin=[]  IntegratorOutMax=[]  FilterOutMin=[]  FilterOutMax=[]  SumI1OutMin=[]  SumI1OutMax=[]  SumI2OutMin=[]  SumI2OutMax=[]  SumI3OutMin=[]  SumI3OutMax=[]  SumI4OutMin=[]  SumI4OutMax=[]  SumDOutMin=[]  SumDOutMax=[]  DifferentiatorOutMin=[]  DifferentiatorOutMax=[]  FilterDiffOutCoefMin=[]  FilterDiffOutCoefMax=[]  ReciprocalOutMin=[]  ReciprocalOutMax=[]  SumDenOutMin=[]  SumDenOutMax=[]  SumNumOutMin=[]  SumNumOutMax=[]  DivideOutMin=[]  DivideOutMax=[]  UdiffTsProdOutMin=[]  UdiffTsProdOutMax=[]  NTsProdOutMin=[]  NTsProdOutMax=[]  UintegralTsProdOutMin=[]  UintegralTsProdOutMax=[]  UngainTsProdOutMin=[]  UngainTsProdOutMax=[]  IntegratorContinuousStateAttributes=''  IntegratorStateMustResolveToSignalObject=off  IntegratorRTWStateStorageClass=Auto  FilterContinuousStateAttributes=''  FilterStateMustResolveToSignalObject=off  FilterRTWStateStorageClass=Auto  ParallelPVariant=Passthrough  IdealPVariant=ExternalParameters  IVariant=ExternalParameters  DVariant=Disabled  IntegratorVariant=Discrete  SatVariant=External  AWVariant=DiscClampingIdeal  PCopyVariant=ExternalParamsIdeal  TRVariant=Disabled  FdbkBlocksVariant=Forward  IdealPFdbkVariant=Disabled  SatFdbkVariant=Disabled  DerivativeFilterVariant=Disabled  NVariant=Disabled  NCopyVariant=Disabled_SignalSpec  FilterICVariant=Disabled  IntegratorICVariant=InternalICs  ExternalResetVariant=Disabled  TRSumVariant=Passthrough  SumFdbkVariant=Disabled  SumVariant=Sum_PI  TsampFilterVariant=InternalTs  TsampNgainVariant=Passthrough  TsampIntegralVariant=Passthrough  ExternalSaturationOutDataTypeStr=Inherit: Same as second input  aMode=0
  Constant : Constant  Value=Aircraft.Control.v_z_up_max  OutDataTypeStr=single
  Constant1 : Constant  Value=Aircraft.Control.v_z_down_max  OutDataTypeStr=single
  Gain : Gain  Gain=-1
  Min : MinMax  Inputs=2
  P_alt : Constant  Value=Aircraft.Control.P_alt  OutDataTypeStr=single
  P_alt1 : Constant  Value=Aircraft.Control.I_alt  OutDataTypeStr=single
  Sum3 : Sum  Inputs=|+-
  ve_z_cmd : Outport
  wires:
  P_alt/1 -> Altitude PID/2
  Sum3/1 -> Altitude PID/1
  max_v_z_mps/1 -> Min/1
  Constant/1 -> Min/2
  Constant1/1 -> Altitude PID/4
  Min/1 -> Gain/1
  Gain/1 -> Altitude PID/5
  P_alt1/1 -> Altitude PID/3
  Altitude PID/1 -> ve_z_cmd/1
  target_z_m/1 -> Sum3/1
  cur_z_m/1 -> Sum3/2

== system double_integrator_sim/WAYPOINT CONTROLLER1/WP_NAV/heading_controller/heading_controller ==
  heading_cmd_rad : Inport
  <heading_rad> : Inport  Port=2
  D_heading : Constant  Value=Aircraft.Control.D_heading  OutDataTypeStr=single
  Discrete Derivative : simulink/Discrete/Discrete Derivative  gainval=1.0  ICPrevScaledInput=0.0  OutMin=[]  OutMax=[]  OutDataType=fixdt(1, 16)  OutScaling=2^-10  DoSatur=off
  I_heading : Constant  Value=Aircraft.Control.I_heading  OutDataTypeStr=single
  PID Controller2 : slpidlib/PID Controller  Controller=PI  Form=Ideal  TimeDomain=Discrete-time  UseExternalTs=off  SampleTime=framePeriod_s  IntegratorMethod=Forward Euler  FilterMethod=Forward Euler  ControllerParametersSource=external  P=1.85  I=0.01  UseKiTs=off  D=0  N=100  UseFilter=off  TunerSelectOption=Transfer Function Based (PID Tuner App)  InitialConditionSource=internal  InitialConditionForIntegrator=0  InitialConditionForFilter=0  DifferentiatorICPrevScaledInput=0  ExternalReset=none  TrackingMode=off  Kt=1  LimitOutput=on  SatLimitsSource=internal  UpperSaturationLimit=inf  LowerSaturationLimit=-inf  LinearizeAsGain=on  AntiWindupMode=clamping  Kb=2  POutMin=[]  POutMax=[]  IOutMin=[]  IOutMax=[]  DOutMin=[]  DOutMax=[]  NOutMin=[]  NOutMax=[]  SumOutMin=[]  SumOutMax=[]  SaturationOutMin=[]  SaturationOutMax=[]  PParamMin=[]  PParamMax=[]  IParamMin=[]  IParamMax=[]  DParamMin=[]  DParamMax=[]  NParamMin=[]  NParamMax=[]  KbParamMin=[]  KbParamMax=[]  KtParamMin=[]  KtParamMax=[]  KbOutMin=[]  KbOutMax=[]  KtOutMin=[]  KtOutMax=[]  IntegratorOutMin=[]  IntegratorOutMax=[]  FilterOutMin=[]  FilterOutMax=[]  SumI1OutMin=[]  SumI1OutMax=[]  SumI2OutMin=[]  SumI2OutMax=[]  SumI3OutMin=[]  SumI3OutMax=[]  SumI4OutMin=[]  SumI4OutMax=[]  SumDOutMin=[]  SumDOutMax=[]  DifferentiatorOutMin=[]  DifferentiatorOutMax=[]  FilterDiffOutCoefMin=[]  FilterDiffOutCoefMax=[]  ReciprocalOutMin=[]  ReciprocalOutMax=[]  SumDenOutMin=[]  SumDenOutMax=[]  SumNumOutMin=[]  SumNumOutMax=[]  DivideOutMin=[]  DivideOutMax=[]  UdiffTsProdOutMin=[]  UdiffTsProdOutMax=[]  NTsProdOutMin=[]  NTsProdOutMax=[]  UintegralTsProdOutMin=[]  UintegralTsProdOutMax=[]  UngainTsProdOutMin=[]  UngainTsProdOutMax=[]  IntegratorContinuousStateAttributes=''  IntegratorStateMustResolveToSignalObject=off  IntegratorRTWStateStorageClass=Auto  FilterContinuousStateAttributes=''  FilterStateMustResolveToSignalObject=off  FilterRTWStateStorageClass=Auto  ParallelPVariant=Passthrough  IdealPVariant=ExternalParameters  IVariant=ExternalParameters  DVariant=Disabled  IntegratorVariant=Discrete  SatVariant=Enabled  AWVariant=DiscClampingIdeal  PCopyVariant=ExternalParamsIdeal  TRVariant=Disabled  FdbkBlocksVariant=Forward  IdealPFdbkVariant=Disabled  SatFdbkVariant=Disabled  DerivativeFilterVariant=Disabled  NVariant=Disabled  NCopyVariant=Disabled_SignalSpec  FilterICVariant=Disabled  IntegratorICVariant=InternalICs  ExternalResetVariant=Disabled  TRSumVariant=Passthrough  SumFdbkVariant=Disabled  SumVariant=Sum_PI  TsampFilterVariant=InternalTs  TsampNgainVariant=Passthrough  TsampIntegralVariant=Passthrough  ExternalSaturationOutDataTypeStr=Inherit: Same as second input  aMode=0
  P_heading : Constant  Value=Aircraft.Control.P_heading  OutDataTypeStr=single
  Product : Product
  Saturation : Saturate  UpperLimit=Aircraft.Control.yaw_rate_max  LowerLimit=-Aircraft.Control.yaw_rate_max
  Sum : Sum  Inputs=|+-
  heading_error : Subsystem
  yaw_rate_cmd : Outport
  wires:
  P_heading/1 -> PID Controller2/2
  heading_cmd_rad/1 -> heading_error/1(heading_cmd_rad)
  I_heading/1 -> PID Controller2/3
  <heading_rad>/1 -> Discrete Derivative/1, heading_error/2(heading_rad)
  Saturation/1 -> yaw_rate_cmd/1
  heading_error/1(heading_error_rad) -> PID Controller2/1
  Discrete Derivative/1 -> Product/1
  D_heading/1 -> Product/2
  PID Controller2/1 -> Sum/1
  Sum/1 -> Saturation/1
  Product/1 -> Sum/2

== system double_integrator_sim/WP_NAV/Horizontal position controller/Horizontal_position_controller/convert to ve_cmd ==
  speed_cmd_mps : Inport
  bearing_to_target_rad : Inport  Port=2
  Cos : Trigonometry  Operator=cos
  Product : Product
  Product1 : Product
  Sin : Trigonometry
  ve_x_cmd : Outport
  ve_y_cmd : Outport  Port=2
  wires:
  Product/1 -> ve_x_cmd/1
  speed_cmd_mps/1 -> Product/1, Product1/1
  bearing_to_target_rad/1 -> Cos/1, Sin/1
  Cos/1 -> Product/2
  Sin/1 -> Product1/2
  Product1/1 -> ve_y_cmd/1

== system double_integrator_sim/WP_NAV/Horizontal position controller/Horizontal_position_controller/convert to ve_cmd1 ==
  speed_cmd_mps : Inport
  bearing_to_target_rad : Inport  Port=2
  Cos : Trigonometry  Operator=cos
  Product : Product
  Product1 : Product
  Sin : Trigonometry
  ve_x_cmd : Outport
  ve_y_cmd : Outport  Port=2
  wires:
  Product/1 -> ve_x_cmd/1
  speed_cmd_mps/1 -> Product/1, Product1/1
  bearing_to_target_rad/1 -> Cos/1, Sin/1
  Cos/1 -> Product/2
  Sin/1 -> Product1/2
  Product1/1 -> ve_y_cmd/1

== system double_integrator_sim/WP_NAV/Horizontal position controller/Horizontal_position_controller/gnd_spd_constraint  ==
  v_e_x_in : Inport
  v_e_y_in : Inport  Port=2
  max_v_hor_mps : Inport  Port=3
  Demux : Demux  Outputs=2
  Magnitude Squared : Math  Operator=magnitude^2
  Mux : Mux  Inputs=2
  Normalization1 : dspmathops/Normalization  NormType=2-norm  Bias=1e-10  NormOver=Each column  Dimension=1  roundingMode=Floor  overflowMode=off  accumDataTypeStr=Inherit: Same as product output  accumLastDataTypeStr=Inherit: Same as product output  outputDataTypeStr=Inherit: Same as product output  outputMin=[]  outputMax=[]  outputLastDataTypeStr=Inherit: Same as product output
  Product : Product
  Sqrt : Sqrt
  Subtract : Sum  Inputs=-+
  Sum of Elements : Sum  Inputs=+
  Switch : Switch  Criteria=u2 > Threshold  SaturateOnIntegerOverflow=off  InputSameDT=off
  v_e_x_out : Outport
  v_e_y_out : Outport  Port=2
  wires:
  Mux/1 -> Magnitude Squared/1, Switch/3, Normalization1/1
  v_e_x_in/1 -> Mux/1
  v_e_y_in/1 -> Mux/2
  Demux/1 -> v_e_x_out/1
  Demux/2 -> v_e_y_out/1
  Switch/1 -> Demux/1
  Product/1 -> Switch/1
  Magnitude Squared/1 -> Sum of Elements/1
  Sum of Elements/1 -> Sqrt/1
  max_v_hor_mps/1 -> Product/2, Subtract/1
  Sqrt/1 -> Subtract/2
  Normalization1/1 -> Product/1
  Subtract/1 -> Switch/2
